simulink model "model"  (R2018a)
settings: Solver=VariableStepAuto  StartTime=0.0  StopTime=10.0  RelTol=1e-3
settings Model: Creator=User  LastModifiedBy=User

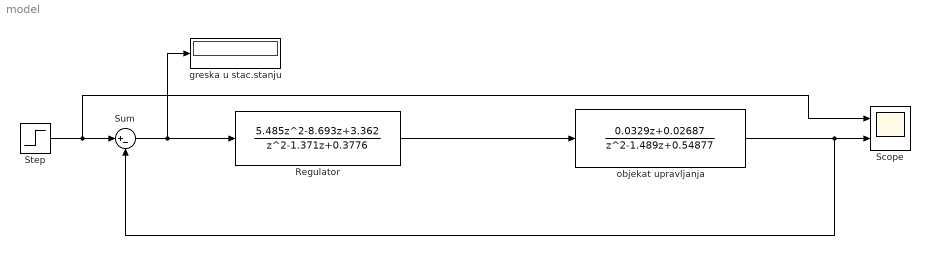
== system model ==
  "Regulator " : DiscreteTransferFcn  Numerator=[5.485 -8.693 3.362]  Denominator=[1 -1.371 0.3776]
  Scope : Scope  NumInputPorts=2
  Step : Step  SampleTime=0
  Sum : Sum  Inputs=|+-
  "greska u stac.stanju " : Display
  "objekat upravljanja " : DiscreteTransferFcn  Numerator=[0.0329 0.02687]  Denominator=[1 -1.489 0.54877]
  wires:
  "Regulator "/1 -> "objekat upravljanja "/1
  Step/1 -> Scope/1, Sum/1
  Sum/1 -> "greska u stac.stanju "/1, "Regulator "/1
  "objekat upravljanja "/1 -> Sum/2, Scope/2
